simulink model "48Vto200V_controller"  (R2026a)
settings: Solver=VariableStepAuto  StopTime=0.5
libraries: slpidlib x1
settings Model: Creator=riddh  LastModifiedBy=riddh

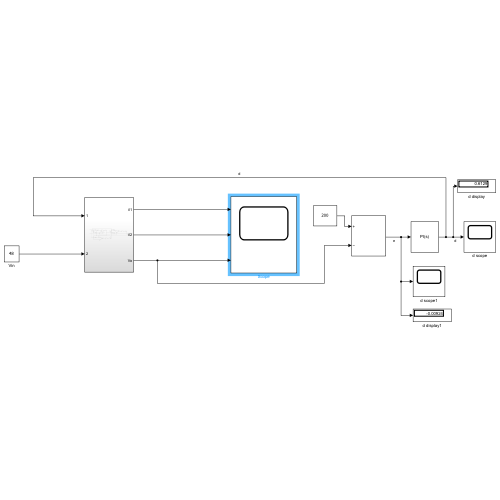
[thumbnail: Simulink's stored preview of the top-level diagram]
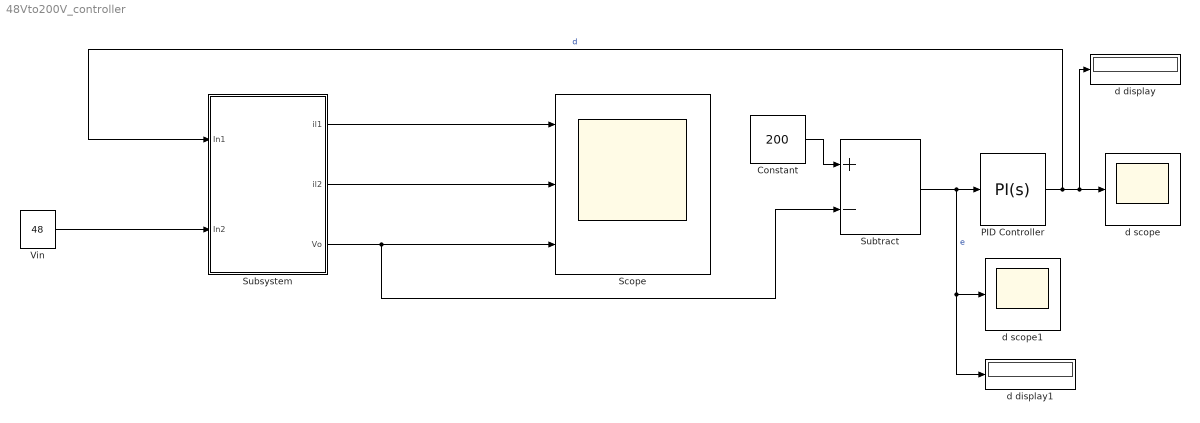
== system 48Vto200V_controller ==
  Constant : Constant  Value=200
  PID Controller : slpidlib/PID Controller  Controller=PI  Form=Parallel  TimeDomain=Continuous-time  UseExternalTs=off  SampleTime=-1  IntegratorMethod=Forward Euler  FilterMethod=Forward Euler  ControllerParametersSource=internal  P=0.0000113  I=0.15288  UseKiTs=off  D=0  UseExternalDerivativeSource=off  N=100  UseFilter=on  TunerSelectOption=Transfer Function Based (PID Tuner App)  InitialConditionSource=internal  InitialConditionForIntegrator=0  InitialConditionForFilter=0  DifferentiatorICPrevScaledInput=0  ExternalReset=none  TrackingMode=off  Kt=1  LimitOutput=off  SatLimitsSource=internal  UpperSaturationLimit=inf  LowerSaturationLimit=-inf  LinearizeAsGain=on  AntiWindupMode=none  Kb=1  LimitIntegrator=off  UpperIntegratorSaturationLimit=inf  LowerIntegratorSaturationLimit=-inf  POutMin=[]  POutMax=[]  IOutMin=[]  IOutMax=[]  DOutMin=[]  DOutMax=[]  NOutMin=[]  NOutMax=[]  SumOutMin=[]  SumOutMax=[]  SaturationOutMin=[]  SaturationOutMax=[]  PParamMin=[]  PParamMax=[]  IParamMin=[]  IParamMax=[]  DParamMin=[]  DParamMax=[]  NParamMin=[]  NParamMax=[]  KbParamMin=[]  KbParamMax=[]  KtParamMin=[]  KtParamMax=[]  KbOutMin=[]  KbOutMax=[]  KtOutMin=[]  KtOutMax=[]  IntegratorOutMin=[]  IntegratorOutMax=[]  FilterOutMin=[]  FilterOutMax=[]  SumI1OutMin=[]  SumI1OutMax=[]  SumI2OutMin=[]  SumI2OutMax=[]  SumI3OutMin=[]  SumI3OutMax=[]  SumI4OutMin=[]  SumI4OutMax=[]  SumDOutMin=[]  SumDOutMax=[]  DifferentiatorOutMin=[]  DifferentiatorOutMax=[]  FilterDiffOutCoefMin=[]  FilterDiffOutCoefMax=[]  ReciprocalOutMin=[]  ReciprocalOutMax=[]  SumDenOutMin=[]  SumDenOutMax=[]  SumNumOutMin=[]  SumNumOutMax=[]  DivideOutMin=[]  DivideOutMax=[]  UdiffTsProdOutMin=[]  UdiffTsProdOutMax=[]  NTsProdOutMin=[]  NTsProdOutMax=[]  UintegralTsProdOutMin=[]  UintegralTsProdOutMax=[]  UngainTsProdOutMin=[]  UngainTsProdOutMax=[]  ClampingZeroOutDataTypeStr=Inherit: Inherit via back propagation  ClampingZeroOutMin=[]  ClampingZeroOutMax=[]  FilterDenConstantOutDataTypeStr=Inherit: Inherit via back propagation  FilterDenConstantOutMin=[]  FilterDenConstantOutMax=[]  PCopyOutDataTypeStr=Inherit: Inherit via back propagation  PCopyOutMin=[]  PCopyOutMax=[]  NCopyOutDataTypeStr=Inherit: Inherit via back propagation  NCopyOutMin=[]  NCopyOutMax=[]  IntegratorContinuousStateAttributes=''  IntegratorStateMustResolveToSignalObject=off  IntegratorRTWStateStorageClass=Auto  FilterContinuousStateAttributes=''  FilterStateMustResolveToSignalObject=off  FilterRTWStateStorageClass=Auto  ParallelPVariant=InternalParameters  IdealPVariant=Disabled  IVariant=InternalParameters  DVariant=Disabled  IntegratorVariant=Continuous  SatVariant=Disabled  AWVariant=Passthrough  PCopyVariant=Disabled  TRVariant=Disabled  FdbkBlocksVariant=Forward  IdealPFdbkVariant=Disabled  SatFdbkVariant=Disabled  DerivativeFilterVariant=Disabled  NVariant=Disabled  NCopyVariant=Disabled_SignalSpec  FilterICVariant=Disabled  IntegratorICVariant=InternalICs  ExternalResetVariant=Disabled  TRSumVariant=Passthrough  SumFdbkVariant=Disabled  SumVariant=Sum_PI  TsampFilterVariant=InternalTs  TsampNgainVariant=Passthrough  TsampIntegralVariant=Disabled_SignalSpec  ExternalSaturationOutDataTypeStr=Inherit: Same as second input  DerivativeSourceVariant=Disabled  PreIntVariant=InternalPreInt
  Scope : Scope  NumInputPorts=3
      settings: ActiveDisplayYMinimum=-13.660318894734207  ActiveDisplayYMaximum=14.587863218041441
  Subsystem : Subsystem
  Subtract : Sum  Inputs=+-
  Vin : Constant  Value=48
  d display : Display
  d display1 : Display
  d scope : Scope
      settings: ActiveDisplayYMinimum=-1  ActiveDisplayYMaximum=1
  d scope1 : Scope
      settings: ActiveDisplayYMinimum=-1  ActiveDisplayYMaximum=1  DataLoggingVariableName=ScopeData2
  wires:
  Vin/1 -> Subsystem/2(In2)
  Subsystem/1(il1) -> Scope/1
  Subsystem/2(il2) -> Scope/2
  Subsystem/3(Vo) -> Subtract/2, Scope/3
  Constant/1 -> Subtract/1
  Subtract/1 -> d display1/1, d scope1/1, PID Controller/1  "e"
  PID Controller/1 -> Subsystem/1(In1), d display/1, d scope/1  "d"

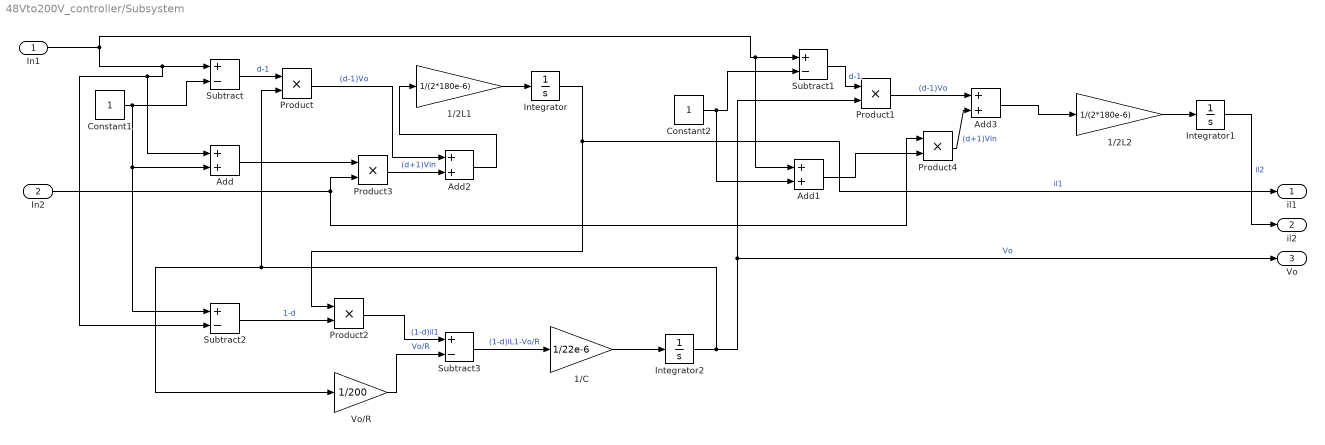
== system 48Vto200V_controller/Subsystem ==
  In1 : Inport
  In2 : Inport  Port=2
  1/2L1 : Gain  Gain=1/(2*180e-6)
  1/2L2 : Gain  Gain=1/(2*180e-6)
  1/C : Gain  Gain=1/22e-6
  Add{,1..3} (4 alike) : Sum
  Constant1 : Constant
  Constant2 : Constant
  Integrator : Integrator
  Integrator1 : Integrator
  Integrator2 : Integrator
  Product{,1..4} (5 alike) : Product
  Subtract{,1..3} (4 alike) : Sum  Inputs=+-
  Vo/R : Gain  Gain=1/200
  il1 : Outport
  il2 : Outport  Port=2
  Vo : Outport  Port=3
  wires:
  Add/1 -> Product3/1
  Vo/R/1 -> Subtract3/2  "Vo/R"
  Product1/1 -> Add3/1  "(d-1)Vo"
  Add2/1 -> 1/2L1/1
  Constant2/1 -> Add1/2, Subtract1/2
  Product2/1 -> Subtract3/1  "(1-d)il1"
  1/C/1 -> Integrator2/1
  Subtract/1 -> Product/1  "d-1"
  Product4/1 -> Add3/2  "(d+1)Vin"
  Product/1 -> Add2/1  "(d-1)Vo"
  Integrator2/1 -> Vo/1, Product1/2, Vo/R/1, Product/2  "Vo"
  Subtract1/1 -> Product1/1  "d-1"
  Add1/1 -> Product4/2
  Integrator/1 -> il1/1, Product2/1  "il1"
  Constant1/1 -> Subtract/2, Add/2, Subtract2/1
  1/2L1/1 -> Integrator/1
  In1/1 -> Subtract/1, Add/1, Subtract2/2, Add1/1, Subtract1/1
  Add3/1 -> 1/2L2/1
  Subtract3/1 -> 1/C/1  "(1-d)iL1-Vo/R"
  Product3/1 -> Add2/2  "(d+1)Vin"
  1/2L2/1 -> Integrator1/1
  In2/1 -> Product4/1, Product3/2
  Subtract2/1 -> Product2/2  "1-d"
  Integrator1/1 -> il2/1  "il2"
